simulink model "malt_indi"  (R2023a)
settings: Solver=FixedStepAuto  StartTime=0.0  StopTime=10.0  FixedStep=0.001  RelTol=1e-3
undefined symbols (not defined in the file or in its folder): framePeriod_s
settings Model: Creator=lagerprocessor  LastModifiedBy=abhandari1
settings DebuggingCC: ParameterPrecisionLossMsg=none

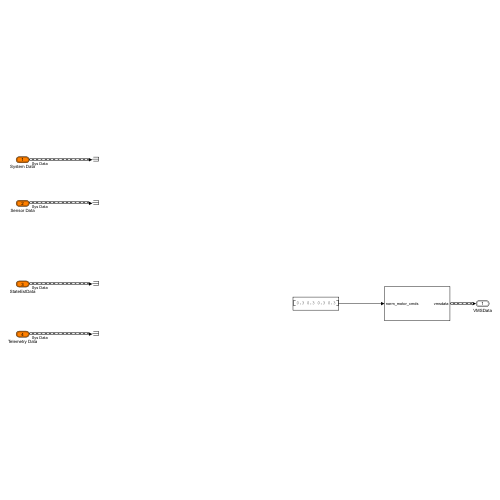
[thumbnail: Simulink's stored preview of the top-level diagram]
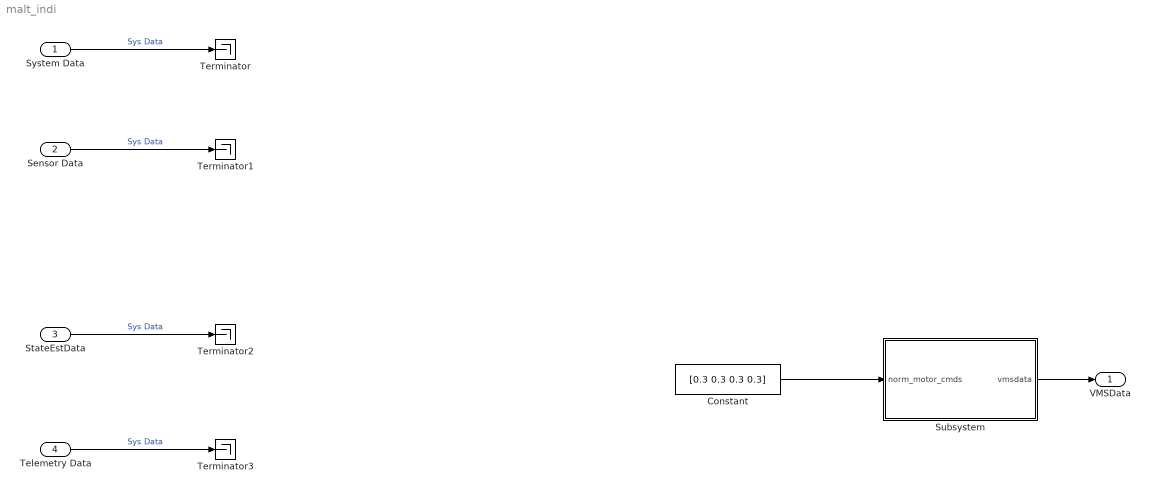
== system malt_indi ==
  System Data : Inport  OutDataTypeStr=Bus: SysData  SampleTime=framePeriod_s  BusOutputAsStruct=on
  Sensor Data : Inport  Port=2  OutDataTypeStr=Bus: SensorData  SampleTime=framePeriod_s  BusOutputAsStruct=on
  StateEstData : Inport  Port=3  OutDataTypeStr=Bus: StateEstData  BusOutputAsStruct=on
  Telemetry Data : Inport  Port=4  OutDataTypeStr=Bus: TelemData  SampleTime=framePeriod_s  BusOutputAsStruct=on
  Constant : Constant  Value=[0.3 0.3 0.3 0.3]  OutDataTypeStr=single
  Subsystem : Subsystem
  Terminator{,1..3} (4 alike) : Terminator
  VMSData : Outport  OutDataTypeStr=Bus: VmsData
  wires:
  Subsystem/1(vmsdata) -> VMSData/1
  Constant/1 -> Subsystem/1(norm_motor_cmds)
  System Data/1 -> Terminator/1  "Sys Data"
  Sensor Data/1 -> Terminator1/1  "Sys Data"
  StateEstData/1 -> Terminator2/1  "Sys Data"
  Telemetry Data/1 -> Terminator3/1  "Sys Data"

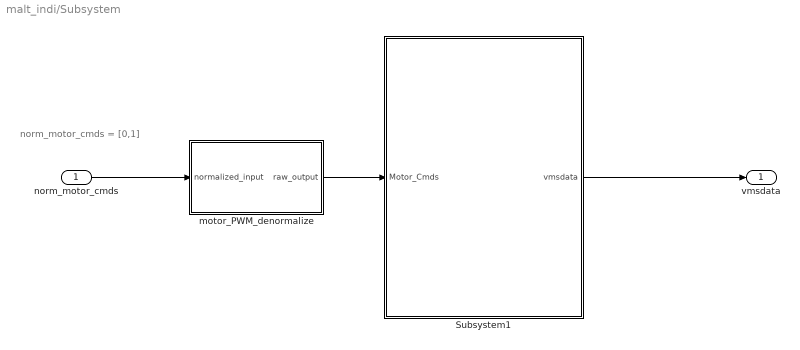
== system malt_indi/Subsystem ==
  note: norm_motor_cmds = [0,1]
  norm_motor_cmds : Inport
  Subsystem1 : Subsystem
  motor_PWM_denormalize : Subsystem
  vmsdata : Outport
  wires:
  motor_PWM_denormalize/1(raw_output) -> Subsystem1/1(Motor_Cmds)
  Subsystem1/1(vmsdata) -> vmsdata/1
  norm_motor_cmds/1 -> motor_PWM_denormalize/1(normalized_input)

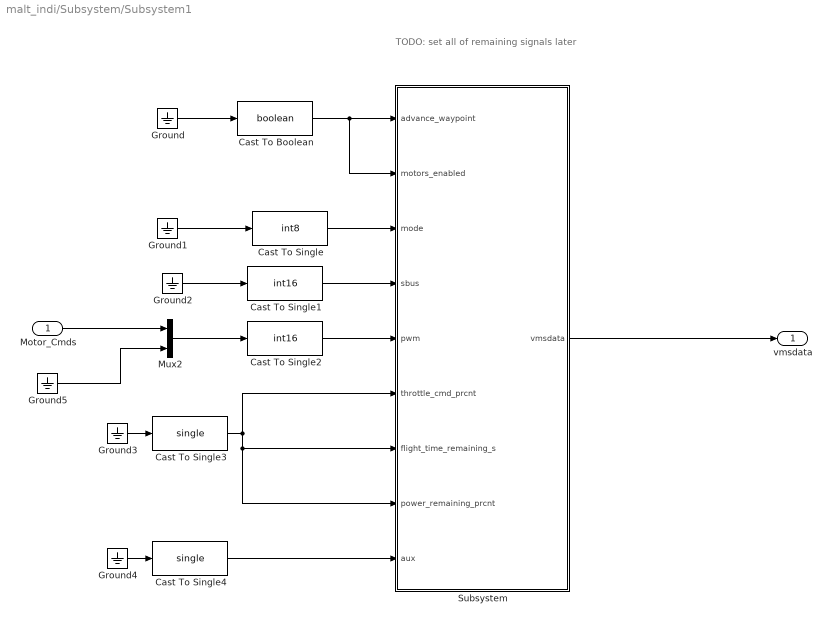
== system malt_indi/Subsystem/Subsystem1 ==
  note: TODO: set all of remaining signals later
  Motor_Cmds : Inport
  Cast To Boolean : DataTypeConversion  OutDataTypeStr=boolean  SaturateOnIntegerOverflow=off  RndMeth=Floor
  Cast To Single : DataTypeConversion  OutDataTypeStr=int8  SaturateOnIntegerOverflow=off  RndMeth=Floor
  Cast To Single1 : DataTypeConversion  OutDataTypeStr=int16  SaturateOnIntegerOverflow=off  RndMeth=Floor
  Cast To Single2 : DataTypeConversion  OutDataTypeStr=int16  SaturateOnIntegerOverflow=off  RndMeth=Floor
  Cast To Single3 : DataTypeConversion  OutDataTypeStr=single  SaturateOnIntegerOverflow=off  RndMeth=Floor
  Cast To Single4 : DataTypeConversion  OutDataTypeStr=single  SaturateOnIntegerOverflow=off  RndMeth=Floor
  Ground{,1..5} (6 alike) : Ground
  Mux2 : Mux  Inputs=2
  Subsystem : Subsystem
  vmsdata : Outport
  wires:
  Cast To Single/1 -> Subsystem/3(mode)
  Ground3/1 -> Cast To Single3/1
  Motor_Cmds/1 -> Mux2/1
  Cast To Single3/1 -> Subsystem/6(throttle_cmd_prcnt), Subsystem/8(power_remaining_prcnt), Subsystem/7(flight_time_remaining_s)
  Ground2/1 -> Cast To Single1/1
  Ground1/1 -> Cast To Single/1
  Cast To Single2/1 -> Subsystem/5(pwm)
  Cast To Single1/1 -> Subsystem/4(sbus)
  Cast To Single4/1 -> Subsystem/9(aux)
  Ground4/1 -> Cast To Single4/1
  Subsystem/1(vmsdata) -> vmsdata/1
  Ground/1 -> Cast To Boolean/1
  Cast To Boolean/1 -> Subsystem/2(motors_enabled), Subsystem/1(advance_waypoint)
  Mux2/1 -> Cast To Single2/1
  Ground5/1 -> Mux2/2

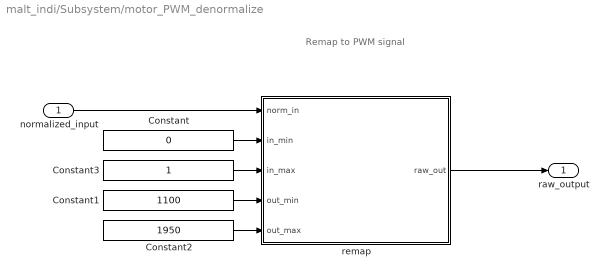
== system malt_indi/Subsystem/motor_PWM_denormalize ==
  note: Remap to PWM signal
  normalized_input : Inport
  Constant : Constant  Value=0  OutDataTypeStr=single
  Constant1 : Constant  Value=1100  OutDataTypeStr=single
  Constant2 : Constant  Value=1950  OutDataTypeStr=single
  Constant3 : Constant  OutDataTypeStr=single
  remap : MATLAB Function  TreatAsAtomicUnit=on
  raw_output : Outport
  wires:
  Constant2/1 -> remap/5(out_max)
  Constant1/1 -> remap/4(out_min)
  Constant3/1 -> remap/3(in_max)
  Constant/1 -> remap/2(in_min)
  remap/1(raw_out) -> raw_output/1
  normalized_input/1 -> remap/1(norm_in)

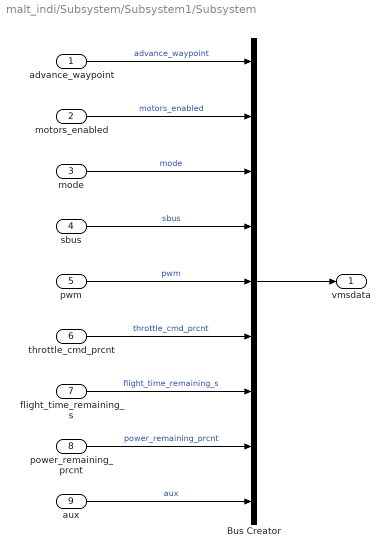
== system malt_indi/Subsystem/Subsystem1/Subsystem ==
  advance_waypoint : Inport
  motors_enabled : Inport  Port=2
  mode : Inport  Port=3
  sbus : Inport  Port=4
  pwm : Inport  Port=5
  throttle_cmd_prcnt : Inport  Port=6
  flight_time_remaining_s : Inport  Port=7
  power_remaining_prcnt : Inport  Port=8
  aux : Inport  Port=9
  Bus Creator : BusCreator  Inputs=9  OutDataTypeStr=Bus: VmsData  NonVirtualBus=on
      settings: InheritFromInputs=off
  vmsdata : Outport
  wires:
  flight_time_remaining_s/1 -> Bus Creator/7  "flight_time_remaining_s"
  mode/1 -> Bus Creator/3  "mode"
  pwm/1 -> Bus Creator/5  "pwm"
  aux/1 -> Bus Creator/9  "aux"
  throttle_cmd_prcnt/1 -> Bus Creator/6  "throttle_cmd_prcnt"
  Bus Creator/1 -> vmsdata/1
  motors_enabled/1 -> Bus Creator/2  "motors_enabled"
  advance_waypoint/1 -> Bus Creator/1  "advance_waypoint"
  power_remaining_prcnt/1 -> Bus Creator/8  "power_remaining_prcnt"
  sbus/1 -> Bus Creator/4  "sbus"

== matlab function malt_indi/Subsystem/motor_PWM_denormalize/remap ==
  data: norm_in input; raw_out output; in_min input; in_max input; out_min input; out_max input
function raw_out = remap(norm_in,in_min,in_max,out_min,out_max)
raw_out = (norm_in - in_min) * (out_max - out_min)/(in_max-in_min) + out_min;
